simulink model "Admittance_Control"  (R2019b)
settings: Solver=VariableStepAuto  StartTime=0.0  StopTime=100  RelTol=1e-3  EnableMultiTasking=on
settings Model: Creator=fanqi  LastModifiedBy=74544
settings DataIOCC: ReturnWorkspaceOutputs=off
settings OptimizationCC: LifeSpan=inf
settings DebuggingCC: SFUnexpectedBacktrackingDiag=warning  SFNoUnconditionalDefaultTransitionDiag=warning  ArithmeticOperatorsInVariantConditions=warning
settings SFSimCC: SimUseLocalCustomCode=off  CustomCodeUndefinedFunction=UseInterfaceOnly
settings RTWCC: RTWUseLocalCustomCode=off
settings CodeAppCC: StateflowObjectComments=on
settings GRTTargetCC: TargetLangStandard=C89/C90 (ANSI)  GeneratePreprocessorConditionals=Disable all
settings ConfigComp: CovMetricSettings=dw  CovHtmlReporting=on  CovSaveCumulativeToWorkspaceVar=on  CovSaveSingleToWorkspaceVar=on  CovExternalEMLEnable=off

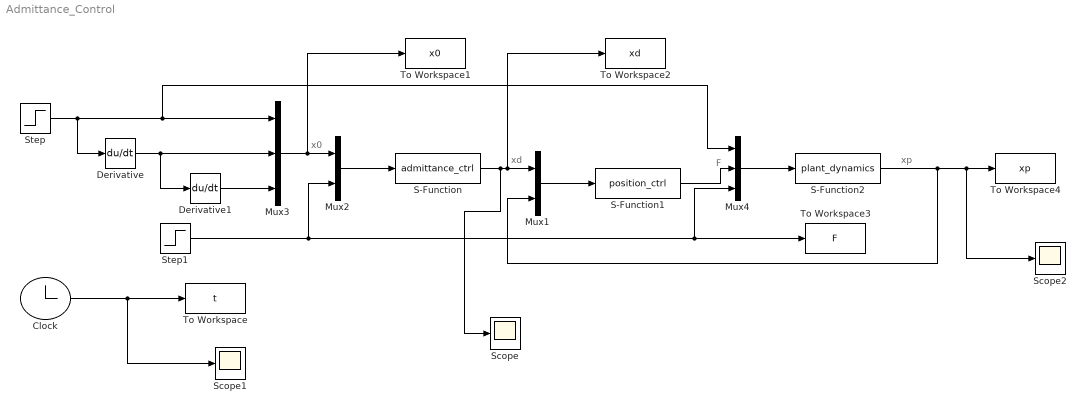
== system Admittance_Control ==
  note: xp
  note: F
  note: xd
  note: x0
  Clock : Clock
      settings: Decimation=50
  Derivative : Derivative
  Derivative1 : Derivative
  Mux1 : Mux  Inputs=2
  Mux2 : Mux  Inputs=2
  Mux3 : Mux  Inputs=3
  Mux4 : Mux  Inputs=3
  S-Function : S-Function  FunctionName=admittance_ctrl  SFunctionDeploymentMode=off  EnableBusSupport=off
  S-Function1 : S-Function  FunctionName=position_ctrl  SFunctionDeploymentMode=off  EnableBusSupport=off
  S-Function2 : S-Function  FunctionName=plant_dynamics  SFunctionDeploymentMode=off  EnableBusSupport=off
  Scope : Scope
  Scope1 : Scope
  Scope2 : Scope
  Step : Step  Time=-0.5  SampleTime=0.001
  Step1 : Step  Time=50  Before=10  After=0  SampleTime=0
  To Workspace : ToWorkspace  VariableName=t  SampleTime=-1
  To Workspace1 : ToWorkspace  VariableName=x0  SampleTime=-1
  To Workspace2 : ToWorkspace  VariableName=xd  SampleTime=-1
  To Workspace3 : ToWorkspace  VariableName=F  SampleTime=-1
  To Workspace4 : ToWorkspace  VariableName=xp  SampleTime=-1
  wires:
  S-Function/1 -> Scope/1, To Workspace2/1, Mux1/1
  Mux1/1 -> S-Function1/1
  S-Function1/1 -> Mux4/2
  S-Function2/1 -> Mux1/2, Scope2/1, To Workspace4/1
  Mux2/1 -> S-Function/1
  Mux3/1 -> To Workspace1/1, Mux2/1
  Clock/1 -> Scope1/1, To Workspace/1
  Step/1 -> Derivative/1, Mux4/1, Mux3/1
  Derivative/1 -> Derivative1/1, Mux3/2
  Derivative1/1 -> Mux3/3
  Mux4/1 -> S-Function2/1
  Step1/1 -> To Workspace3/1, Mux4/3, Mux2/2
